simulink model "ProyectoFinal"  (R2025a)
settings: Solver=ode8  StartTime=0.0  StopTime=inf  FixedStep=0.01  RelTol=1e-3
undefined symbols (not defined in the file or in its folder): CR, DiscIntNeverNeededParam, LF
libraries: simulink x4, instrumentseriallib x4, spsRMSLib x1
settings Model: PacingRate=1000  Creator=aceve  LastModifiedBy=sergio2416

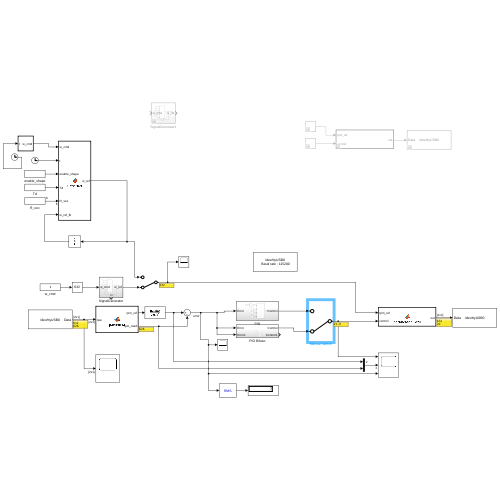
[thumbnail: Simulink's stored preview of the top-level diagram]
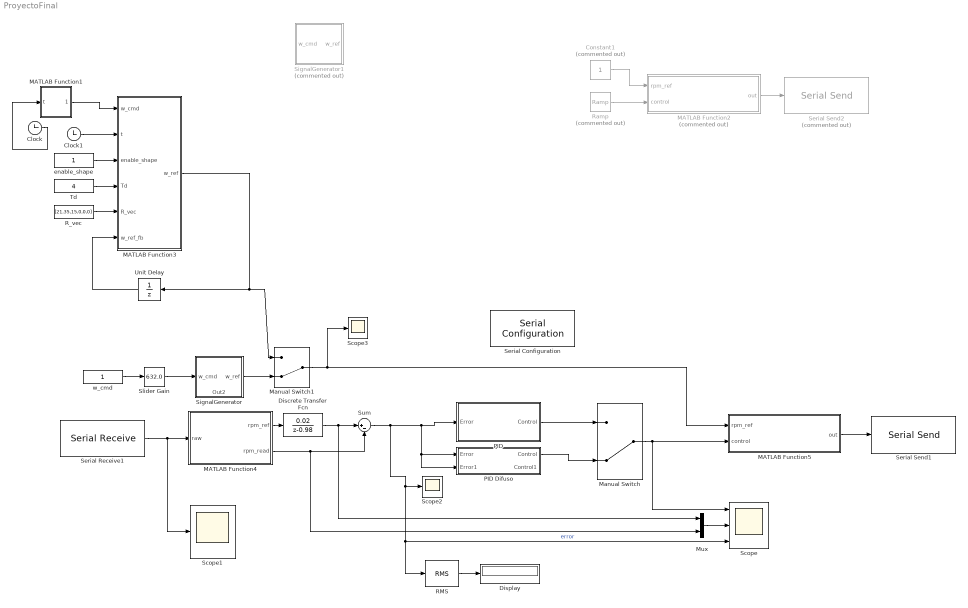
== system ProyectoFinal ==
  Clock : Clock
  Clock1 : Clock
  Constant1 : Constant  Commented=on
  Discrete Transfer Fcn : DiscreteTransferFcn  Numerator=[0.02]  Denominator=[1 -0.98]
  Display : Display
  MATLAB Function1 : MATLAB Function  TreatAsAtomicUnit=on
  MATLAB Function2 : MATLAB Function  Commented=on  TreatAsAtomicUnit=on
  MATLAB Function3 : MATLAB Function  TreatAsAtomicUnit=on
  MATLAB Function4 : MATLAB Function  TreatAsAtomicUnit=on
  MATLAB Function5 : MATLAB Function  TreatAsAtomicUnit=on
  Manual Switch : ManualSwitch  CurrentSetting=0
  Manual Switch1 : ManualSwitch  CurrentSetting=0
  Mux : Mux  Inputs=2
  PID : Subsystem
  PID Difuso : Subsystem
  RMS : spsRMSLib/RMS  TrueRMS=on  Freq=60  RMSInit=120  Ts=0
  R_vec : Constant  Value=[21,35,15,0,0,0]  SampleTime=-1
  Ramp : simulink/Sources/Ramp  Commented=on  slope=0.5  start=0  InitialOutput=20
  Scope : Scope  NumInputPorts=3
      settings: ActiveDisplayYMinimum=16.25  ActiveDisplayYMaximum=53.75
  Scope1 : Scope
      settings: ActiveDisplayYMinimum=-8157.7499999999982  ActiveDisplayYMaximum=73439.75
  Scope2 : Scope
      settings: ActiveDisplayYMinimum=552.25  ActiveDisplayYMaximum=1049.75  DataLoggingVariableName=ScopeData2
  Scope3 : Scope
      settings: ActiveDisplayYMinimum=-1  ActiveDisplayYMaximum=1  DataLoggingVariableName=ScopeData3
  Serial Configuration : instrumentseriallib/Serial Configuration  Priority=-200000  PortSel=/dev/ttyUSB0  Port=/dev/ttyUSB0  ComPort=/dev/ttyUSB0  BaudRate=115200  DataBits=8  Parity=none  StopBits=1  ByteOrder=little-endian  FlowControl=none  Timeout=10  SimulateUsing=Interpreted execution  BlockInModel=on  aMode=1
  Serial Receive1 : instrumentseriallib/Serial Receive  Priority=1  PortSel=/dev/ttyUSB0  Port=/dev/ttyUSB0  ComPort=/dev/ttyUSB0  DataType=uint16  SaveDataType=uint8  ToggleHeader=off  Header=[]  ToggleDataSize=on  DataSize=[2 1]  ToggleTerminator=off  Terminator=CR/LF ('\r\n')  CustomTerminator=[]  InputFormat=Column major  EnableBlockingMode=on  ActionDataUnavailable=Output last received value  ActionWhenDataUnavailable=Output last received value  CustomValue=0  SampleTime=0.01  SimulateUsing=Interpreted execution  BlockInModel=on  aMode=1  LibraryInUse=instrumentlib
  Serial Send1 : instrumentseriallib/Serial Send  Priority=1  PortSel=/dev/ttyUSB0  Port=/dev/ttyUSB0  ComPort=/dev/ttyUSB0  Header=[]  Terminator=<none>  CustomTerminator=[]  EnableBlockingMode=off  SimulateUsing=Interpreted execution  BlockInModel=on  aMode=1
  Serial Send2 : instrumentseriallib/Serial Send  Priority=1  Commented=on  PortSel=/dev/ttyUSB0  Port=/dev/ttyUSB0  ComPort=/dev/ttyUSB0  Header=[]  Terminator=<none>  CustomTerminator=[]  EnableBlockingMode=off  SimulateUsing=Interpreted execution  BlockInModel=on  aMode=1
  SignalGenerator : Subsystem
      settings: PortSchema="{\"entries\":[{\"content\":{\"sides\":[{\"content\":{\"connectorIds\":[\"In1\"]},\"type\":\"ConnectorPlacement.EquallySpacedRectSide\",\"uuid\":\"4cce06af-7d16-41fd-b2cd-3f9504ea5661\"},{\"content\":{\"connectorIds\":[\"Out1\"],\"side\":\"RIGHT\"},\"type\":\"ConnectorPlacement.EquallySpacedRectSide\",\"uuid\":\"e46f2018-f9b0-4466-8f5a-c2ac3a5d4f95\"},{\"content\":{\"side\":\"TOP\"},\"type\":\"ConnectorPlacement.EquallySpacedRectSide\",\"uuid\":\"729f40e1-48e2-4108-bf21-b45cfb3ac552\"},{\"content\":{\"connectorIds\":[\"Out2\"],\"side\":\"BOTTOM\"},\"type\":\"ConnectorPlacement.EquallySpacedRectSide\",\"uuid\":\"bad99237-78e2-4514-a1cb-77583f4be541\"}]},\"type\":\"ConnectorPlacement.EquallySpacedConnector\",\"uuid\":\"bd502931-cf11-490a-aa85-e71776c8b5bf\"}],\"packageUris\":[\"http://schema.mathworks.com/mf0/Connector/R2020b\"],\"version\":\"1.0\"}"
  SignalGenerator1 : Subsystem  Commented=on
  Slider Gain : simulink/Math Operations/Slider Gain  gain=632.0  low=500  high=1100
  Sum : Sum  Inputs=|+-
  Td : Constant  Value=4  SampleTime=-1
  Unit Delay : UnitDelay  SampleTime=-1  HasFrameUpgradeWarning=on
  enable_shape : Constant  SampleTime=-1
  w_cmd : Constant  SampleTime=-1
  wires:
  Sum/1 -> PID/1(Error), PID Difuso/2(Error1), PID Difuso/1(Error), RMS/1, Scope/3, Scope2/1  "error"
  w_cmd/1 -> Slider Gain/1
  Serial Receive1/1 -> Scope1/1, MATLAB Function4/1(raw)
  MATLAB Function5/1(out) -> Serial Send1/1
  Manual Switch/1 -> Scope/1, MATLAB Function5/2(control)
  Slider Gain/1 -> SignalGenerator/1(w_cmd)
  MATLAB Function2/1(out) -> Serial Send2/1
  Ramp/1 -> MATLAB Function2/2(control)
  Constant1/1 -> MATLAB Function2/1(rpm_ref)
  Mux/1 -> Scope/2
  RMS/1 -> Display/1
  enable_shape/1 -> MATLAB Function3/3(enable_shape)
  Td/1 -> MATLAB Function3/4(Td)
  Unit Delay/1 -> MATLAB Function3/6(w_ref_fb)
  Clock/1 -> MATLAB Function1/1(t)
  R_vec/1 -> MATLAB Function3/5(R_vec)
  Clock1/1 -> MATLAB Function3/2(t)
  MATLAB Function1/1(w_cmd) -> MATLAB Function3/1(w_cmd)
  MATLAB Function4/2(rpm_read) -> Mux/2, Sum/2
  PID/1(Control) -> Manual Switch/1
  SignalGenerator/1(w_ref) -> Manual Switch1/2
  MATLAB Function3/1(w_ref) -> Manual Switch1/1, Unit Delay/1
  Manual Switch1/1 -> Scope3/1, MATLAB Function5/1(rpm_ref)
  MATLAB Function4/1(rpm_ref) -> Discrete Transfer Fcn/1
  Discrete Transfer Fcn/1 -> Mux/1, Sum/1
  PID Difuso/1(Control) -> Manual Switch/2

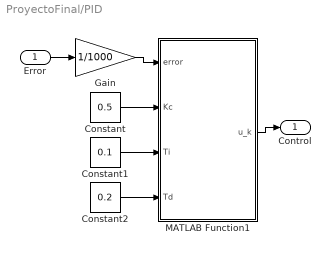
== system ProyectoFinal/PID ==
  Error : Inport
  Constant : Constant  Value=0.5
  Constant1 : Constant  Value=0.1
  Constant2 : Constant  Value=0.2
  Gain : Gain  Gain=1/1000
  MATLAB Function1 : MATLAB Function  TreatAsAtomicUnit=on
  Control : Outport
  wires:
  Gain/1 -> MATLAB Function1/1(error)
  Error/1 -> Gain/1
  MATLAB Function1/1(u_k) -> Control/1
  Constant/1 -> MATLAB Function1/2(Kc)
  Constant2/1 -> MATLAB Function1/4(Td)
  Constant1/1 -> MATLAB Function1/3(Ti)

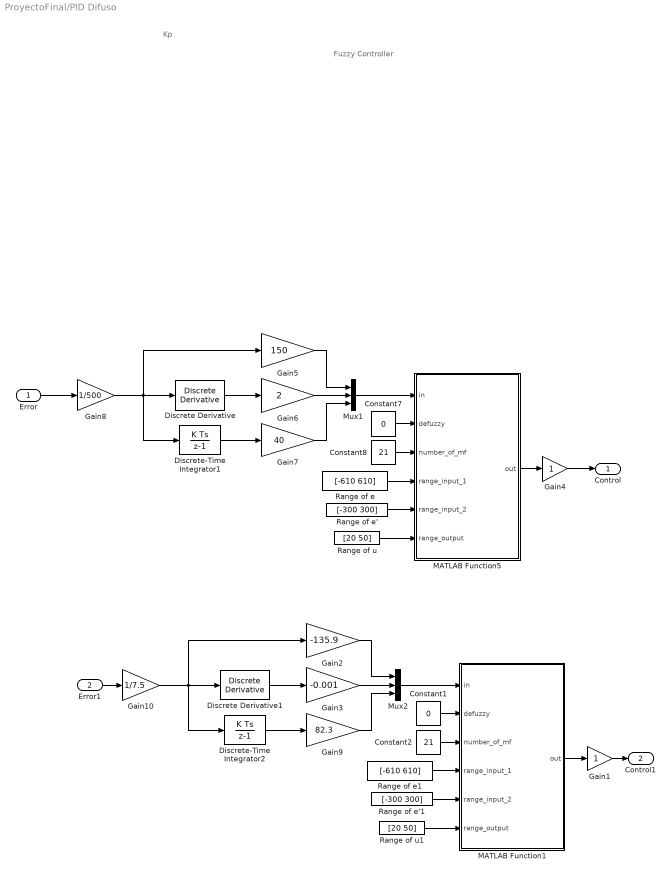
== system ProyectoFinal/PID Difuso ==
  note: Fuzzy Controller
  note: Kp
  Error : Inport
  Error1 : Inport  Port=2
  Constant1 : Constant  Value=0
  Constant2 : Constant  Value=21
  Constant7 : Constant  Value=0
  Constant8 : Constant  Value=21
  Discrete Derivative : simulink/Discrete/Discrete Derivative  gainval=1.0  ICPrevScaledInput=0.0  OutMin=[]  OutMax=[]  OutDataType=fixdt(1, 16)  OutScaling=2^-10  DoSatur=off
  Discrete Derivative1 : simulink/Discrete/Discrete Derivative  gainval=1.0  ICPrevScaledInput=0.0  OutMin=[]  OutMax=[]  OutDataType=fixdt(1, 16)  OutScaling=2^-10  DoSatur=off
  Discrete-Time Integrator1 : DiscreteIntegrator  SampleTime=0.01  LimitOutput=on  UpperSaturationLimit=65  LowerSaturationLimit=0  ICPrevOutput=DiscIntNeverNeededParam  ICPrevScaledInput=DiscIntNeverNeededParam
  Discrete-Time Integrator2 : DiscreteIntegrator  SampleTime=0.01  LimitOutput=on  UpperSaturationLimit=65  LowerSaturationLimit=0  ICPrevOutput=DiscIntNeverNeededParam  ICPrevScaledInput=DiscIntNeverNeededParam
  Gain1 : Gain
  Gain10 : Gain  Gain=1/7.5
  Gain2 : Gain  Gain=-135.9
  Gain3 : Gain  Gain=-0.001
  Gain4 : Gain
  Gain5 : Gain  Gain=150
  Gain6 : Gain  Gain=2
  Gain7 : Gain  Gain=40
  Gain8 : Gain  Gain=1/500
  Gain9 : Gain  Gain=82.3
  MATLAB Function1 : MATLAB Function  TreatAsAtomicUnit=on
  MATLAB Function5 : MATLAB Function  TreatAsAtomicUnit=on
  Mux1 : Mux  Inputs=3
  Mux2 : Mux  Inputs=3
  Range of e : Constant  Value=[-610 610]
  Range of e' : Constant  Value=[-300 300]
  Range of e'1 : Constant  Value=[-300 300]
  Range of e1 : Constant  Value=[-610 610]
  Range of u : Constant  Value=[20 50]
  Range of u1 : Constant  Value=[20 50]
  Control : Outport
  Control1 : Outport  Port=2
  wires:
  Gain7/1 -> Mux1/3
  Range of e/1 -> MATLAB Function5/4(range_input_1)
  Gain8/1 -> Discrete-Time Integrator1/1, Gain5/1, Discrete Derivative/1
  Gain6/1 -> Mux1/2
  MATLAB Function5/1(out) -> Gain4/1
  Constant8/1 -> MATLAB Function5/3(number_of_mf)
  Mux1/1 -> MATLAB Function5/1(in)
  Discrete Derivative/1 -> Gain6/1
  Discrete-Time Integrator1/1 -> Gain7/1
  Range of e'/1 -> MATLAB Function5/5(range_input_2)
  Range of u/1 -> MATLAB Function5/6(range_output)
  Constant7/1 -> MATLAB Function5/2(defuzzy)
  Gain5/1 -> Mux1/1
  Gain4/1 -> Control/1
  Error/1 -> Gain8/1
  Gain2/1 -> Mux2/1
  Range of e1/1 -> MATLAB Function1/4(range_input_1)
  Range of e'1/1 -> MATLAB Function1/5(range_input_2)
  Mux2/1 -> MATLAB Function1/1(in)
  MATLAB Function1/1(out) -> Gain1/1
  Gain9/1 -> Mux2/3
  Constant1/1 -> MATLAB Function1/2(defuzzy)
  Gain3/1 -> Mux2/2
  Gain10/1 -> Discrete-Time Integrator2/1, Gain2/1, Discrete Derivative1/1
  Range of u1/1 -> MATLAB Function1/6(range_output)
  Constant2/1 -> MATLAB Function1/3(number_of_mf)
  Discrete Derivative1/1 -> Gain3/1
  Discrete-Time Integrator2/1 -> Gain9/1
  Error1/1 -> Gain10/1
  Gain1/1 -> Control1/1

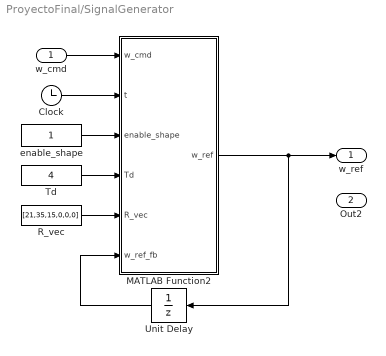
== system ProyectoFinal/SignalGenerator ==
  w_cmd : Inport
  Clock : Clock
  MATLAB Function2 : MATLAB Function  TreatAsAtomicUnit=on
  R_vec : Constant  Value=[21,35,15,0,0,0]  SampleTime=-1
  Td : Constant  Value=4  SampleTime=-1
  Unit Delay : UnitDelay  SampleTime=-1  HasFrameUpgradeWarning=on
  enable_shape : Constant  SampleTime=-1
  w_ref : Outport
  Out2 : Outport  Port=2
  wires:
  Clock/1 -> MATLAB Function2/2(t)
  Td/1 -> MATLAB Function2/4(Td)
  enable_shape/1 -> MATLAB Function2/3(enable_shape)
  Unit Delay/1 -> MATLAB Function2/6(w_ref_fb)
  R_vec/1 -> MATLAB Function2/5(R_vec)
  MATLAB Function2/1(w_ref) -> Unit Delay/1, w_ref/1
  w_cmd/1 -> MATLAB Function2/1(w_cmd)

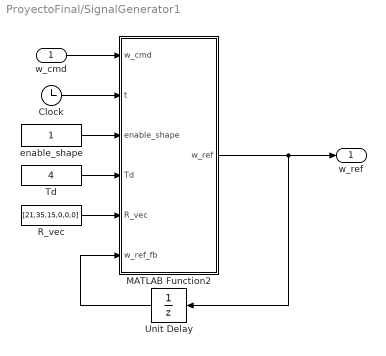
== system ProyectoFinal/SignalGenerator1 ==
  w_cmd : Inport
  Clock : Clock
  MATLAB Function2 : MATLAB Function  TreatAsAtomicUnit=on
  R_vec : Constant  Value=[21,35,15,0,0,0]  SampleTime=-1
  Td : Constant  Value=4  SampleTime=-1
  Unit Delay : UnitDelay  SampleTime=-1  HasFrameUpgradeWarning=on
  enable_shape : Constant  SampleTime=-1
  w_ref : Outport
  wires:
  Clock/1 -> MATLAB Function2/2(t)
  Td/1 -> MATLAB Function2/4(Td)
  enable_shape/1 -> MATLAB Function2/3(enable_shape)
  Unit Delay/1 -> MATLAB Function2/6(w_ref_fb)
  R_vec/1 -> MATLAB Function2/5(R_vec)
  MATLAB Function2/1(w_ref) -> Unit Delay/1, w_ref/1
  w_cmd/1 -> MATLAB Function2/1(w_cmd)

== matlab function ProyectoFinal/MATLAB Function5 ==
  data: rpm_ref input; control input; out output
function out = packRefAndPWM(rpm_ref, control)
% Esta función ahora empaqueta [rpm_ref, frequency_hz]
% El 'control_signal' (antes 'voltage') viene de 0-60 desde el "Knob".

% --- 1. Escalado lineal ---
% Frecuencia (0-60 Hz)
target_freq = control;

% --- 2. Empaquetado ---
% Convierte ambos valores a uint16 para enviar por UART
freq_u16 = uint16(target_freq);
rpm_ref_u16 = uint16(rpm_ref);

% El ESP32 espera recibir: [rpm_ref, frecuencia_en_hz]
out = uint16([rpm_ref_u16, freq_u16]);

end

== matlab function ProyectoFinal/PID Difuso/MATLAB Function1 ==
  data: in input; out output; defuzzy input; number_of_mf input; range_input_1 input; range_input_2 input; range_output input
function out = fcn(in, defuzzy, number_of_mf, range_input_1, range_input_2, range_output)
% CONTROLADOR FUZZY PID (Fuzzy PD + I + Bias)
% =========================================================
% Entradas (in):
%   in(1): Error (Escalado por K_fp)
%   in(2): Derivada del Error (Escalado por K_fd)
%   in(3): Acción Integral (Escalado por K_fi)
%
% Parámetros:
%   defuzzy: 0 = COG (Centroide), 1 = CA (Promedio)
%   range_output: [min, max] (Ej: [20, 55])
% =========================================================

% --- 1. PREPARACIÓN DE DIVISIONES (UNIVERSOS) ---
n = number_of_mf;

% Universos de Entrada (Tal cual vienen de los parámetros)
div1 = linspace(range_input_1(1), range_input_1(2), n); % Error
div2 = linspace(range_input_2(1), range_input_2(2), n); % d_Error

% --- UNIVERSO DE SALIDA CENTRADO (LA CLAVE DEL ÉXITO) ---
% Calculamos el ancho total del rango de salida (Ej: 55 - 20 = 35)
ancho = range_output(2) - range_output(1);
mitad = ancho / 2.0;

% Creamos un universo simétrico centrado en 0 (Ej: de -17.5 a +17.5).
% Esto asegura que si Error=0, la salida difusa (corrección) sea 0.
div_out = linspace(-mitad, mitad, n);


% --- 2. FUZZIFICACIÓN (Calcular Membresías) ---
mu_e  = compute_memberships(in(1), div1);
mu_de = compute_memberships(in(2), div2);


% --- 3. DEFINIR FAM (Reglas Diagonales para PD) ---
% Crea una matriz diagonal típica de control (Negativo-Cero-Positivo)
FAM = zeros(n, n);
middle_val = (n + 1) / 2;
middle_ij = middle_val*2;

for i = 1:n
    for j = 1:n
        v = middle_val + middle_ij - (i + j);
        % Saturar índices por seguridad
        if v > n, v = n; end
        if v < 1, v = 1; end
        FAM(i,j) = v;
    end
end


% --- 4. INFERENCIA (Activación de Reglas) ---
rule_heights = zeros(n,n);
for i = 1:n
    for j = 1:n
        % Método del Mínimo (Mamdani)
        rule_heights(i,j) = min(mu_e(i), mu_de(j));
    end
end

% Agregación: Máxima activación por etiqueta de salida
mu_out = zeros(1,n);
for k = 1:n
    mask = (FAM == k);
    if any(mask(:))
        mu_out(k) = max(rule_heights(mask));
    else
        mu_out(k) = 0;
    end
end


% --- 5. DEFUZZIFICACIÓN (Calcular Salida PD) ---
% output: fuzzy_pd_out (será un valor cercano a 0 si no hay error)

% Valor por defecto: Centro exacto (0)
midL = floor((n+1)/2);
midR = ceil((n+1)/2);
fuzzy_pd_out = 0.5*(div_out(midL) + div_out(midR)); 

if defuzzy == 0
    % --- COG (Centro de Gravedad / Centroide) ---
    num = 0; den = 0;
    if n > 1
        step = div_out(2)-div_out(1);
    else
        step = 1; % Seguridad
    end
    base = 2*step; % Ancho base de los triángulos
    
    for k = 1:n
        h = mu_out(k);
        if h > 0
            % Área de un trapecio truncado por h
            top_base = (1-h)*base;
            A = h*(base+top_base)/2;
            
            num = num + A*div_out(k);
            den = den + A;
        end
    end
    if den > eps
        fuzzy_pd_out = num/den;
    end
    
else
    % --- CA (Promedio Ponderado de Alturas) ---
    num = sum(mu_out .* div_out);
    den = sum(mu_out);
    if den > eps
        fuzzy_pd_out = num/den;
    end
end


% --- 6. COMBINACIÓN FINAL (PD + I + BIAS) ---
% AQUI ESTÁ EL TRUCO PARA ELIMINAR EL PICO INICIAL:
% 1. fuzzy_pd_out: Corrección dinámica (aprox 0 en equilibrio)
% 2. in(3): Integral (Corrección de error estacionario)
% 3. 22.0: BIAS FIJO (Energía base para mantener 540 RPM)

out_unclamped = fuzzy_pd_out + in(3) + 17.04;


% --- 7. SATURACIÓN DE SEGURIDAD ---
% Forzamos a que nunca salga del rango físico [20, 55]
if out_unclamped < range_output(1)
    out = range_output(1);
elseif out_unclamped > range_output(2)
    out = range_output(2);
else
    out = out_unclamped;
end

end

% =========================================================
% FUNCIONES AUXILIARES
% =========================================================
function mu = compute_memberships(x, div)
    % Calcula la membresía triangular para una entrada x
    % sobre un vector de divisiones 'div'
    n = length(div);
    mu = zeros(1,n);
    
    % Fuera de rango izquierdo
    if x <= div(1)
        mu(1) = 1; return
    end
    % Fuera de rango derecho
    if x >= div(end)
        mu(end) = 1; return
    end
    
    % Buscar intervalo
    for i = 1:n-1
        x1 = div(i); 
        x2 = div(i+1);
        
        if x >= x1 && x <= x2
            den = x2 - x1;
            if den == 0, den = eps; end
            
            % Triángulo izquierdo (subida)
            mu(i+1) = (x - x1)/den;
            % Triángulo derecho (bajada)
            mu(i)   = (x2 - x)/den;
            return
        end
    end
end

== matlab function ProyectoFinal/MATLAB Function2 ==
  data: rpm_ref input; control input; out output
function out = packRefAndPWM(rpm_ref, control)
% Esta función ahora empaqueta [rpm_ref, frequency_hz]
% El 'control_signal' (antes 'voltage') viene de 0-60 desde el "Knob".

% --- 1. Define la escala de la SEÑAL DE CONTROL ---
control_min = 20;
control_max = 60;

% --- 2. Define la escala de la FRECUENCIA de salida ---
freq_min = 20;     % Frecuencia mínima (0 Hz = motor detenido)
freq_max = 60;    % Frecuencia máxima (ej. 60 Hz)

% --- 3. Escalado lineal ---
% Convierte la señal de control (0-60) a frecuencia (0-60 Hz)
target_freq = (control - control_min) * (freq_max - freq_min) / (control_max - control_min) + freq_min;

% --- 4. Saturación ---
% Asegura que la frecuencia esté dentro de los límites
if target_freq > freq_max
    target_freq = freq_max;
elseif target_freq < freq_min
    target_freq = freq_min;
end

% --- 5. Empaquetado ---
% Convierte ambos valores a uint16 para enviar por UART
freq_u16 = uint16(target_freq);
rpm_ref_u16 = uint16(rpm_ref);

% El ESP32 espera recibir: [rpm_ref, frecuencia_en_hz]
out = uint16([rpm_ref_u16, freq_u16]);

end

== matlab function ProyectoFinal/PID/MATLAB Function1 ==
  data: error input; u_k output; Kc input; Ti input; Td input
function u_k = PID(error, Kc, Ti, Td)
% PID discreto con salida escalada de 0–1 a 20–50
% Entradas:
%   error : e(k)
%   Kc    : ganancia proporcional
%   Ti    : tiempo integral
%   Td    : tiempo derivativo

% Parámetros internos
Ts = 0.005;   % Tiempo de muestreo (constante)
N  = 100;    % Filtro derivativo (constante)

persistent e_prev i_prev d_prev
if isempty(e_prev)
    e_prev = 0;
    i_prev = 0;
    d_prev = 0;
end

% ----- PID en rango 0–1 -----
p = Kc * error;

i = i_prev + (Kc * Ts / Ti) * error;

c1 = 1 / (1 + Ts * N);
c2 = (Kc * Td * N) / (1 + Ts * N);

d = c1 * d_prev + c2 * (error - e_prev);

u_total = p + i + d;

% Saturación en [0,1]
u_01 = min(max(u_total, 0), 1);

% Actualización de estados
i_prev = i;
d_prev = d;
e_prev = error;

% ----- Mapeo final a rango [20,50] -----
u_k = 20 + u_01 * 30;   % (50 - 20) = 30

end

== matlab function ProyectoFinal/SignalGenerator1/MATLAB Function2 ==
  settings: updateMethod=DISCRETE
  data: w_cmd input; t input; w_ref output; enable_shape input; Td input; R_vec input; w_ref_fb input
function w_ref = BezierRef(w_cmd, t, enable_shape, Td, R_vec, w_ref_fb)
% =================================================================
% VERSIÓN 6 (Corrección de arranque en cero)
% =================================================================
%
% Entradas:
%   w_cmd     : setpoint deseado (de la GUI)
%   t         : tiempo absoluto (Clock)
%   enable_shape : 1 = perfilar, 0 = paso directo
%   Td        : duración de la transición [s]
%   R_vec     : [r1..r6] coeficientes del polinomio
%   w_ref_fb  : w_ref anterior (feedback vía Memory/Unit Delay)
%
% Salida:
%   w_ref     : referencia suavizada

% --- estados persistentes ---
persistent w0 wf t0 last_cmd is_initialized

% --- Lógica de inicialización en el primer paso de ejecución ---
if isempty(is_initialized) || t == 0 % Se reinicia si el tiempo es 0
    is_initialized = true; 
    
    % --- CORRECCIÓN AQUÍ ---
    % Antes decía: w0 = w_ref_fb; (Esto tomaba el 0 del Unit Delay)
    % Ahora dice:
    w0 = w_cmd;  % Forzamos a que el punto de partida sea el comando actual (540)
    wf = w_cmd;
    
    t0 = t;
    last_cmd = w_cmd;
end

% --- FIX 1: Detecta cambio de comando con tolerancia ---
if abs(w_cmd - last_cmd) > 1e-6
    % AQUÍ SÍ usamos w_ref_fb, porque queremos una curva suave desde
    % donde nos quedamos anteriormente.
    w0 = w_ref_fb;
    wf = w_cmd;
    t0 = t;
    last_cmd = w_cmd;
end

% Paso directo si está desactivado
if enable_shape == 0 || Td <= 0
    w_ref = w_cmd;
    w0 = w_cmd; 
    wf = w_cmd;
    last_cmd = w_cmd;
    return
end

% Progreso normalizado en [0,1]
s = (t - t0) / Td;

if s <= 0
    alpha = 0;
elseif s >= 1
    alpha = 1;
else
    % Bezier polinómico
    if numel(R_vec) < 6
        alpha = s; % Fallback a rampa lineal
    else
        r1 = R_vec(1); r2 = R_vec(2); r3 = R_vec(3);
        r4 = R_vec(4); r5 = R_vec(5); r6 = R_vec(6);
        
        % Validación de coeficientes
        if abs((r1 - r2 + r3 - r4 + r5 - r6) - 1.0) > 1e-3
            alpha = s^5;
        else
            alpha = (s.^5).*(r1 - r2*s + r3*s.^2 - r4*s.^3 + r5*s.^4 - r6*s.^5);
        end
    end
    
    % Clampeo por seguridad numérica
    if alpha < 0, alpha = 0; end
    if alpha > 1, alpha = 1; end
end

% Interpolación entre w0 y wf
w_ref = w0 + alpha*(wf - w0);
end

== matlab function ProyectoFinal/SignalGenerator/MATLAB Function2 ==
  settings: updateMethod=DISCRETE
  data: w_cmd input; t input; w_ref output; enable_shape input; Td input; R_vec input; w_ref_fb input
function w_ref = BezierRef(w_cmd, t, enable_shape, Td, R_vec, w_ref_fb)
% =================================================================
% VERSIÓN ANTERIOR (Arranca desde w_ref_fb, usualmente 0)
% =================================================================
%
% Entradas:
%   w_cmd     : setpoint deseado
%   t         : tiempo absoluto
%   enable_shape : 1 = perfilar, 0 = paso directo
%   Td        : duración de la transición [s]
%   R_vec     : [r1..r6] coeficientes
%   w_ref_fb  : valor anterior (Feedback del Unit Delay)

persistent w0 wf t0 last_cmd is_initialized

% --- INICIALIZACIÓN ---
% Aquí es donde ocurre el arranque en 0.
if isempty(is_initialized) || t == 0 
    is_initialized = true; 
    
    % ALERTA: Esto toma el valor del Unit Delay. 
    % Si el Delay inicia en 0, la curva empezará en 0.
    w0 = w_ref_fb; 
    
    wf = w_cmd;
    t0 = t;
    last_cmd = w_cmd;
end

% --- Detecta cambio de comando ---
if abs(w_cmd - last_cmd) > 1e-6
    w0 = w_ref_fb;
    wf = w_cmd;
    t0 = t;
    last_cmd = w_cmd;
end

% Paso directo si está desactivado
if enable_shape == 0 || Td <= 0
    w_ref = w_cmd;
    w0 = w_cmd; 
    wf = w_cmd;
    last_cmd = w_cmd;
    return
end

% Progreso normalizado s en [0,1]
s = (t - t0) / Td;

if s <= 0
    alpha = 0;
elseif s >= 1
    alpha = 1;
else
    % Bezier polinómico
    if numel(R_vec) < 6
        alpha = s; 
    else
        r1 = R_vec(1); r2 = R_vec(2); r3 = R_vec(3);
        r4 = R_vec(4); r5 = R_vec(5); r6 = R_vec(6);
        
        % Validación simple de coeficientes
        if abs((r1 - r2 + r3 - r4 + r5 - r6) - 1.0) > 1e-3
            alpha = s^5;
        else
            alpha = (s.^5).*(r1 - r2*s + r3*s.^2 - r4*s.^3 + r5*s.^4 - r6*s.^5);
        end
    end
    
    % Clampeo
    if alpha < 0, alpha = 0; end
    if alpha > 1, alpha = 1; end
end

% Interpolación
w_ref = w0 + alpha*(wf - w0);

end

== matlab function ProyectoFinal/MATLAB Function1 ==
  data: t input; w_cmd output
function w_cmd = Generador_Perfil(t)
    % Genera la señal escalón para alimentar al suavizador Bezier
    % Secuencia: 540 -> 1160 -> 800
    
    % --- CONFIGURACIÓN DE TIEMPOS ---
    % Td es 4 segundos. Dejamos un margen para que se estabilice.
    t_inicio = 10;   % Tiempo para el primer cambio (540 -> 1160)
    t_bajada = 20;  % Tiempo para el segundo cambio (1160 -> 800)
    
    % --- LÓGICA DE COMANDO ---
    if t < t_inicio
        % Estado inicial
        w_cmd = 600;
        
    elseif t >= t_inicio && t < t_bajada
        % Primer escalón: Subida
        w_cmd = 1160;
        
    else
        % Segundo escalón: Bajada
        w_cmd = 800;
    end
end

== matlab function ProyectoFinal/MATLAB Function4 ==
  data: rpm_ref output; rpm_read output; raw input
function [rpm_ref, rpm_read] = parseRPM(raw)
%#codegen
% raw: 1x2 uint16 vector received from ESP32
% rpm_read: measured RPM from encoder
% rpm_ref:  reference RPM echoed back from ESP32

rpm_read = double(raw(2));   % first  uint16 from ESP32
rpm_ref  = double(raw(1));   % second uint16 from ESP32
end

== matlab function ProyectoFinal/MATLAB Function3 ==
  settings: updateMethod=DISCRETE
  data: w_cmd input; t input; w_ref output; enable_shape input; Td input; R_vec input; w_ref_fb input
function w_ref = BezierRef(w_cmd, t, enable_shape, Td, R_vec, w_ref_fb)
% =================================================================
% VERSIÓN 6 (Corrección de arranque en cero)
% =================================================================
%
% Entradas:
%   w_cmd     : setpoint deseado (de la GUI)
%   t         : tiempo absoluto (Clock)
%   enable_shape : 1 = perfilar, 0 = paso directo
%   Td        : duración de la transición [s]
%   R_vec     : [r1..r6] coeficientes del polinomio
%   w_ref_fb  : w_ref anterior (feedback vía Memory/Unit Delay)
%
% Salida:
%   w_ref     : referencia suavizada

% --- estados persistentes ---
persistent w0 wf t0 last_cmd is_initialized

% --- Lógica de inicialización en el primer paso de ejecución ---
if isempty(is_initialized) || t == 0 % Se reinicia si el tiempo es 0
    is_initialized = true; 
    
    % --- CORRECCIÓN AQUÍ ---
    % Antes decía: w0 = w_ref_fb; (Esto tomaba el 0 del Unit Delay)
    % Ahora dice:
    w0 = w_cmd;  % Forzamos a que el punto de partida sea el comando actual (540)
    wf = w_cmd;
    
    t0 = t;
    last_cmd = w_cmd;
end

% --- FIX 1: Detecta cambio de comando con tolerancia ---
if abs(w_cmd - last_cmd) > 1e-6
    % AQUÍ SÍ usamos w_ref_fb, porque queremos una curva suave desde
    % donde nos quedamos anteriormente.
    w0 = w_ref_fb;
    wf = w_cmd;
    t0 = t;
    last_cmd = w_cmd;
end

% Paso directo si está desactivado
if enable_shape == 0 || Td <= 0
    w_ref = w_cmd;
    w0 = w_cmd; 
    wf = w_cmd;
    last_cmd = w_cmd;
    return
end

% Progreso normalizado en [0,1]
s = (t - t0) / Td;

if s <= 0
    alpha = 0;
elseif s >= 1
    alpha = 1;
else
    % Bezier polinómico
    if numel(R_vec) < 6
        alpha = s; % Fallback a rampa lineal
    else
        r1 = R_vec(1); r2 = R_vec(2); r3 = R_vec(3);
        r4 = R_vec(4); r5 = R_vec(5); r6 = R_vec(6);
        
        % Validación de coeficientes
        if abs((r1 - r2 + r3 - r4 + r5 - r6) - 1.0) > 1e-3
            alpha = s^5;
        else
            alpha = (s.^5).*(r1 - r2*s + r3*s.^2 - r4*s.^3 + r5*s.^4 - r6*s.^5);
        end
    end
    
    % Clampeo por seguridad numérica
    if alpha < 0, alpha = 0; end
    if alpha > 1, alpha = 1; end
end

% Interpolación entre w0 y wf
w_ref = w0 + alpha*(wf - w0);
end

== matlab function ProyectoFinal/PID Difuso/MATLAB Function5 ==
  data: in input; out output; defuzzy input; number_of_mf input; range_input_1 input; range_input_2 input; range_output input
function out = fcn(in, defuzzy, number_of_mf, range_input_1, range_input_2, range_output)
% CONTROLADOR FUZZY PID (Fuzzy PD + I + Bias)
% =========================================================
% Entradas (in):
%   in(1): Error (Escalado por K_fp)
%   in(2): Derivada del Error (Escalado por K_fd)
%   in(3): Acción Integral (Escalado por K_fi)
%
% Parámetros:
%   defuzzy: 0 = COG (Centroide), 1 = CA (Promedio)
%   range_output: [min, max] (Ej: [20, 55])
% =========================================================

% --- 1. PREPARACIÓN DE DIVISIONES (UNIVERSOS) ---
n = number_of_mf;

% Universos de Entrada (Tal cual vienen de los parámetros)
div1 = linspace(range_input_1(1), range_input_1(2), n); % Error
div2 = linspace(range_input_2(1), range_input_2(2), n); % d_Error

% --- UNIVERSO DE SALIDA CENTRADO (LA CLAVE DEL ÉXITO) ---
% Calculamos el ancho total del rango de salida (Ej: 55 - 20 = 35)
ancho = range_output(2) - range_output(1);
mitad = ancho / 2.0;

% Creamos un universo simétrico centrado en 0 (Ej: de -17.5 a +17.5).
% Esto asegura que si Error=0, la salida difusa (corrección) sea 0.
div_out = linspace(-mitad, mitad, n);


% --- 2. FUZZIFICACIÓN (Calcular Membresías) ---
mu_e  = compute_memberships(in(1), div1);
mu_de = compute_memberships(in(2), div2);


% --- 3. DEFINIR FAM (Reglas Diagonales para PD) ---
% Crea una matriz diagonal típica de control (Negativo-Cero-Positivo)
FAM = zeros(n, n);
middle_val = (n + 1) / 2;
middle_ij = middle_val*2;

for i = 1:n
    for j = 1:n
        v = middle_val + middle_ij - (i + j);
        % Saturar índices por seguridad
        if v > n, v = n; end
        if v < 1, v = 1; end
        FAM(i,j) = v;
    end
end


% --- 4. INFERENCIA (Activación de Reglas) ---
rule_heights = zeros(n,n);
for i = 1:n
    for j = 1:n
        % Método del Mínimo (Mamdani)
        rule_heights(i,j) = min(mu_e(i), mu_de(j));
    end
end

% Agregación: Máxima activación por etiqueta de salida
mu_out = zeros(1,n);
for k = 1:n
    mask = (FAM == k);
    if any(mask(:))
        mu_out(k) = max(rule_heights(mask));
    else
        mu_out(k) = 0;
    end
end


% --- 5. DEFUZZIFICACIÓN (Calcular Salida PD) ---
% output: fuzzy_pd_out (será un valor cercano a 0 si no hay error)

% Valor por defecto: Centro exacto (0)
midL = floor((n+1)/2);
midR = ceil((n+1)/2);
fuzzy_pd_out = 0.5*(div_out(midL) + div_out(midR)); 

if defuzzy == 0
    % --- COG (Centro de Gravedad / Centroide) ---
    num = 0; den = 0;
    if n > 1
        step = div_out(2)-div_out(1);
    else
        step = 1; % Seguridad
    end
    base = 2*step; % Ancho base de los triángulos
    
    for k = 1:n
        h = mu_out(k);
        if h > 0
            % Área de un trapecio truncado por h
            top_base = (1-h)*base;
            A = h*(base+top_base)/2;
            
            num = num + A*div_out(k);
            den = den + A;
        end
    end
    if den > eps
        fuzzy_pd_out = num/den;
    end
    
else
    % --- CA (Promedio Ponderado de Alturas) ---
    num = sum(mu_out .* div_out);
    den = sum(mu_out);
    if den > eps
        fuzzy_pd_out = num/den;
    end
end


% --- 6. COMBINACIÓN FINAL (PD + I + BIAS) ---
% AQUI ESTÁ EL TRUCO PARA ELIMINAR EL PICO INICIAL:
% 1. fuzzy_pd_out: Corrección dinámica (aprox 0 en equilibrio)
% 2. in(3): Integral (Corrección de error estacionario)
% 3. 22.0: BIAS FIJO (Energía base para mantener 540 RPM)

out_unclamped = fuzzy_pd_out + in(3) + 20.5;


% --- 7. SATURACIÓN DE SEGURIDAD ---
% Forzamos a que nunca salga del rango físico [20, 55]
if out_unclamped < range_output(1)
    out = range_output(1);
elseif out_unclamped > range_output(2)
    out = range_output(2);
else
    out = out_unclamped;
end

end

% =========================================================
% FUNCIONES AUXILIARES
% =========================================================
function mu = compute_memberships(x, div)
    % Calcula la membresía triangular para una entrada x
    % sobre un vector de divisiones 'div'
    n = length(div);
    mu = zeros(1,n);
    
    % Fuera de rango izquierdo
    if x <= div(1)
        mu(1) = 1; return
    end
    % Fuera de rango derecho
    if x >= div(end)
        mu(end) = 1; return
    end
    
    % Buscar intervalo
    for i = 1:n-1
        x1 = div(i); 
        x2 = div(i+1);
        
        if x >= x1 && x <= x2
            den = x2 - x1;
            if den == 0, den = eps; end
            
            % Triángulo izquierdo (subida)
            mu(i+1) = (x - x1)/den;
            % Triángulo derecho (bajada)
            mu(i)   = (x2 - x)/den;
            return
        end
    end
end
